simulink model "final"  (R2013a)
settings: Solver=VariableStepDiscrete  StartTime=0.0  StopTime=0.1  MaxStep=1e-5  RelTol=1e-3
undefined symbols (not defined in the file or in its folder): dfilt
libraries: dsparch4 x3
settings Model: Creator=cory  LastModifiedBy=cory

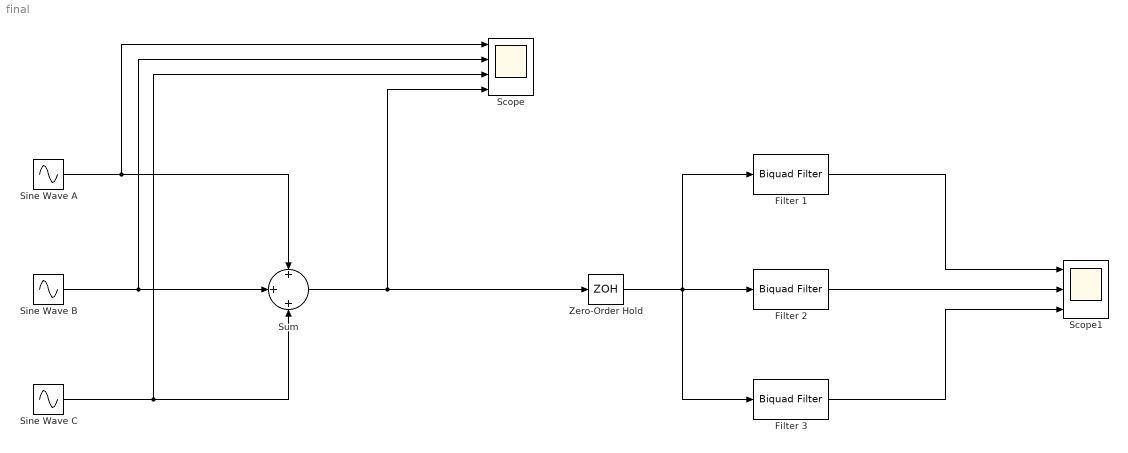
== system final ==
  Filter 1 : dsparch4/Biquad Filter  Tag=BlockMethodSubSystem  IIRFiltStruct=Direct form II  CoeffSource=Specify via dialog  BiQuadCoeffs=[1 -0.95283293913422362 1 1 -1.1259316670360957 0.93629487856096338;1 -0.76558794394961827 1 1 -1.1817650747096444 0.84553663777251609;1 -0.19143863320137666 1 1 -1.2869269559567975 0.68877446776273055;1 1.405522715515706 1 1 -1.3964345467436945 0.52808469942507863;1 -1.0119247183282249 1 1 -1.1103692090404258 0.98314509353382196]  a0Flag=Warning  IC=0  ICnum=0  ICden=0  InputProcessing=Columns as channels (frame based)  denAccumFracLength=30  denProdOutputFracLength=30  secondMemoryFracLength=15  roundingMode=Floor  overflowMode=off  ScaleValues=[0.86159491573695868;0.81683349333787381;0.66703756727848984;0.80498393673654445;0.0080709820598665483;1]  optimizeScaleValues=on  ScaleValueMode=Specify via input port (g)  scaleValueFracLength=14  FilterSource=Specify via dialog  dfiltObjectName=dfilt.df2tsos([1 0.3 0.4],[1 0.1 0.2])
  Filter 2 : dsparch4/Biquad Filter  Tag=BlockMethodSubSystem  IIRFiltStruct=Direct form II  CoeffSource=Specify via dialog  BiQuadCoeffs=[1 -0.44890304834288369 1 1 -0.91933473648994379 0.96934402809904152;1 -1.2722723760091084 1 1 -0.86911636602808195 0.96890213648083989;1 -0.72233518192252255 1 1 -0.96040024520614531 0.9883966952324329;1 -1.076612114443765 1 1 -0.84380035187548752 0.98800371790827712]  a0Flag=Warning  IC=0  ICnum=0  ICden=0  InputProcessing=Columns as channels (frame based)  denAccumFracLength=30  denProdOutputFracLength=30  secondMemoryFracLength=15  roundingMode=Floor  overflowMode=off  ScaleValues=[0.33285428087334418;0.33285428087334418;0.089753534972130983;0.089753534972130983;1]  optimizeScaleValues=on  ScaleValueMode=Specify via input port (g)  scaleValueFracLength=14  FilterSource=Specify via dialog  dfiltObjectName=dfilt.df2tsos([1 0.3 0.4],[1 0.1 0.2])
  Filter 3 : dsparch4/Biquad Filter  Tag=BlockMethodSubSystem  IIRFiltStruct=Direct form II  CoeffSource=Specify via dialog  BiQuadCoeffs=[1 -0.89491165558750152 1 1 -0.35064235646200276 0.83680040820907176;1 -1.2809003066569766 1 1 0.027827946997489039 0.58055843727616119;1 -1.8717747187761302 1 1 0.59368522473455709 0.20736715105893014;1 -0.7515791872796963 1 1 -0.49994762717968666 0.95872126483202325]  a0Flag=Warning  IC=0  ICnum=0  ICden=0  InputProcessing=Columns as channels (frame based)  denAccumFracLength=30  denProdOutputFracLength=30  secondMemoryFracLength=15  roundingMode=Floor  overflowMode=off  ScaleValues=[0.99347999157066447;1.2567088326587721;2.9720385954467625;0.013185830143014443;1]  optimizeScaleValues=on  ScaleValueMode=Specify via input port (g)  scaleValueFracLength=14  FilterSource=Specify via dialog  dfiltObjectName=dfilt.df2tsos([1 0.3 0.4],[1 0.1 0.2])
  Scope : Scope  NumInputPorts=4
      settings: YMin=-5~-5~-5~-5  YMax=5~5~5~5
  Scope1 : Scope  NumInputPorts=3
      settings: YMin=-5~-5~-5  YMax=5~5~5
  Sine Wave A : Sin  Amplitude=2.5  Frequency=2*pi*1500  Phase=pi/2  SampleTime=0
  Sine Wave B : Sin  Amplitude=1.75  Frequency=1750*2*pi  Phase=pi/4  SampleTime=0
  Sine Wave C : Sin  Amplitude=1.25  Frequency=2*pi*2200  Phase=3*pi/4  SampleTime=0
  Sum : Sum  Inputs=+|+|+
  Zero-Order Hold : ZeroOrderHold  SampleTime=1/10000
  wires:
  Sum/1 -> Zero-Order Hold/1, Scope/4
  Sine Wave A/1 -> Scope/1, Sum/1
  Sine Wave B/1 -> Scope/2, Sum/2
  Sine Wave C/1 -> Scope/3, Sum/3
  Zero-Order Hold/1 -> Filter 2/1, Filter 3/1, Filter 1/1
  Filter 1/1 -> Scope1/1
  Filter 2/1 -> Scope1/2
  Filter 3/1 -> Scope1/3
